simulink library "INT_FlSys_DetFlTnk"  (R2016b)
settings: Solver=VariableStepAuto  StartTime=0.0  StopTime=10.0  RelTol=1e-3
settings Model: Creator=zhoutinglin  LastModifiedBy=zhoutinglin

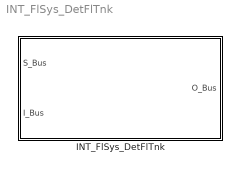
== system INT_FlSys_DetFlTnk ==
  INT_FlSys_DetFlTnk : Subsystem

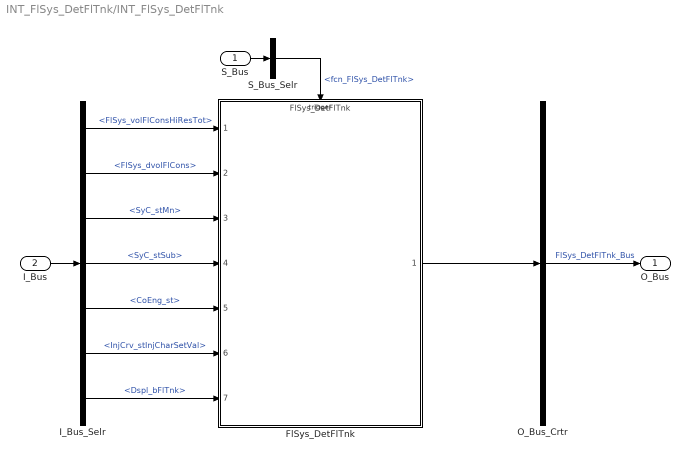
== system INT_FlSys_DetFlTnk/INT_FlSys_DetFlTnk ==
  S_Bus : Inport
  I_Bus : Inport  Port=2
  FlSys_DetFlTnk : ModelReference  ModelNameDialog=FlSys_DetFlTnk  SimulationMode=Normal  ModelReferenceVersion=1.12  TriggerPortName=function  TriggerPortTriggerType=function-call  TriggerPortStatesWhenEnabling=held
  I_Bus_Selr : BusSelector  OutputSignals=FlSys_volFlConsHiResTot,FlSys_dvolFlCons,SyC_stMn,SyC_stSub,CoEng_st,InjCrv_stInjCharSetVal,Dspl_bFlTnk
  O_Bus_Crtr : BusCreator  Inputs=1
  S_Bus_Selr : BusSelector  OutputSignals=fcn_FlSys_DetFlTnk
  O_Bus : Outport
  wires:
  S_Bus_Selr/1 -> FlSys_DetFlTnk/Trigger  "<fcn_FlSys_DetFlTnk>"
  S_Bus/1 -> S_Bus_Selr/1
  I_Bus/1 -> I_Bus_Selr/1
  I_Bus_Selr/1 -> FlSys_DetFlTnk/1  "<FlSys_volFlConsHiResTot>"
  I_Bus_Selr/2 -> FlSys_DetFlTnk/2  "<FlSys_dvolFlCons>"
  I_Bus_Selr/3 -> FlSys_DetFlTnk/3  "<SyC_stMn>"
  I_Bus_Selr/4 -> FlSys_DetFlTnk/4  "<SyC_stSub>"
  I_Bus_Selr/5 -> FlSys_DetFlTnk/5  "<CoEng_st>"
  I_Bus_Selr/6 -> FlSys_DetFlTnk/6  "<InjCrv_stInjCharSetVal>"
  I_Bus_Selr/7 -> FlSys_DetFlTnk/7  "<Dspl_bFlTnk>"
  O_Bus_Crtr/1 -> O_Bus/1  "FlSys_DetFlTnk_Bus"
  FlSys_DetFlTnk/1 -> O_Bus_Crtr/1
